simulink model "k1vistst"  (Simulink 8.5)
settings: Solver=ode45  StartTime=0.0  StopTime=10.0  RelTol=1e-3
libraries: cdsCDI64 x2, cdsCDO64 x2, cdsEpicsBinIn x2, cdsAdcx0 x1, dac x1, TYPEBP_MASTER x1, cdsBit2Word x1, cdsWord2Bit x1, cdsParameters x1
settings Model: Creator=keiko  LastModifiedBy=controls
settings DataIOCC: SignalLoggingSaveFormat=Dataset
settings OptimizationCC: ExpressionDepthLimit=128
settings DebuggingCC: UnderspecifiedInitializationDetection=Simplified  MergeDetectMultiDrivingBlocksExec=error  SolverPrmCheckMsg=warning  FcnCallInpInsideContextMsg=EnableAllAsError  StateNameClashWarn=none
settings GRTTargetCC: CombineOutputUpdateFcns=on  GRTInterface=off

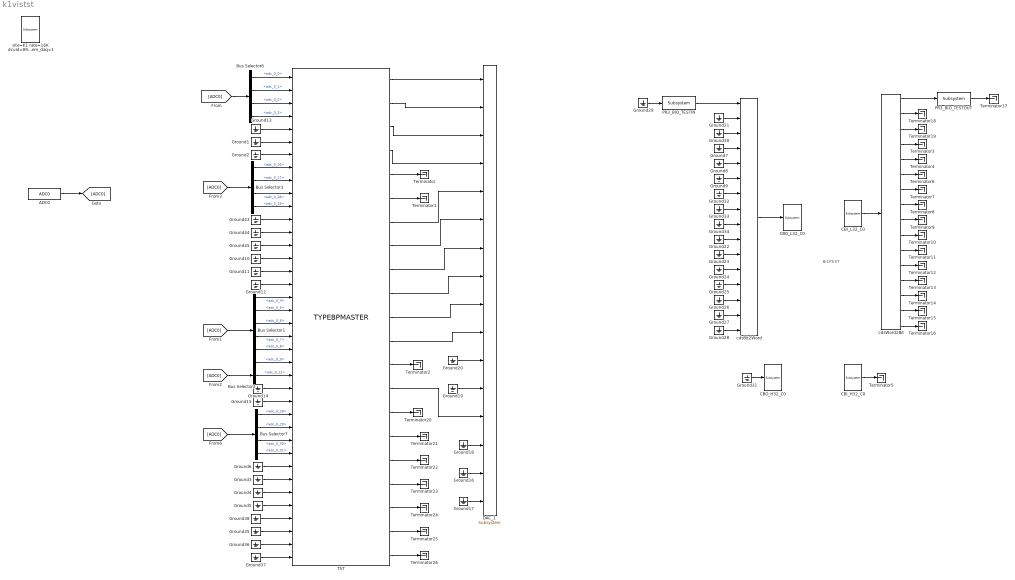
== system k1vistst ==
  note: BIOTEST
  ADC0 : cdsAdcx0/ADC0  Tag=cdsAdc  Description=|
      | type-GSC_16AI64SSA
      | card_num=0
      settings: AttributesFormatString=%<Description>\n%<Tag>
  Bus Selector1 : BusSelector  Description=ADC Selector  OutputSignals=adc_0_4,adc_0_5,adc_0_6,adc_0_7,adc_0_8,adc_0_9
      settings: AttributesFormatString=%<Description>
  Bus Selector2 : BusSelector  Description=ADC Selector  OutputSignals=adc_0_12
      settings: AttributesFormatString=%<Description>
  Bus Selector3 : BusSelector  Description=ADC Selector  OutputSignals=adc_0_16,adc_0_17,adc_0_18,adc_0_19
      settings: AttributesFormatString=%<Description>
  Bus Selector6 : BusSelector  Description=ADC Selector  OutputSignals=adc_0_0,adc_0_1,adc_0_2,adc_0_3
      settings: AttributesFormatString=%<Description>
  Bus Selector7 : BusSelector  Description=ADC Selector  OutputSignals=adc_0_28,adc_0_29,adc_0_30,adc_0_31
      settings: AttributesFormatString=%<Description>
  CBI_H32_C0 : cdsCDI64/Subsystem  Tag=cdsCDI64  Description=card_num=1
      settings: AttributesFormatString=%<Tag>\n%<Description>
  CBI_L32_C0 : cdsCDI64/Subsystem  Tag=cdsCDI64  Description=card_num=0
      settings: AttributesFormatString=%<Tag>\n%<Description>
  CBO_H32_C0 : cdsCDO64/Subsystem  Tag=cdsCDO64  Description=card_num=1
      settings: AttributesFormatString=%<Tag>\n%<Description>
  CBO_L32_C0 : cdsCDO64/Subsystem  Tag=cdsCDO64  Description=card_num=0
      settings: AttributesFormatString=%<Tag>\n%<Description>
  DAC_1 : dac/Subsystem  Description=|
      | type=GSC_16AO16,
      | card_num=0
      settings: AttributesFormatString=%<Description>
  Ground{1..38,43..45} (41 alike) : Ground
  PR3_BIO_TESTIN : cdsEpicsBinIn/Subsystem  Tag=cdsEpicsBinIn  Description=|
      | Purpose:                                                                            
      | Create an EPICS binary (0 or 1) input channel to the FE realtime controls.          
      |                                                                                     
      | Operation:                                                                          
      | Outputs value from an EPICS ai record. Value is binary input (bi Epics record type).
      |                                                                                     
      | Usage:                                                                              
      | Name the part with the desired EPICS channel name.
      settings: AttributesFormatString=%<Tag>
  PR3_BIO_TESTOUT : cdsEpicsBinIn/Subsystem  Tag=cdsEpicsBinIn  Description=|
      | Purpose:                                                                            
      | Create an EPICS binary (0 or 1) input channel to the FE realtime controls.          
      |                                                                                     
      | Operation:                                                                          
      | Outputs value from an EPICS ai record. Value is binary input (bi Epics record type).
      |                                                                                     
      | Usage:                                                                              
      | Name the part with the desired EPICS channel name.
      settings: AttributesFormatString=%<Tag>
  TST : TYPEBP_MASTER/TYPEBPMASTER
      settings: AttributesFormatString=%<Description>
  Terminator{,1..26} (27 alike) : Terminator
  cdsBit2Word : cdsBit2Word/cdsBit2Word  Tag=cdsBit2Word  Description=Forms single 16 bit integer from 16 0/1 inputs.
      settings: AttributesFormatString=%<Tag>
  cdsWord2Bit : cdsWord2Bit/cdsWord2Bit  Tag=cdsWord2Bit  Description=Generate 16 0/1 outputs from single 16-bit integer input
      settings: AttributesFormatString=cdsWord2Bit
  site=K1 rate=16K dcuid=89 host=k1pr0 specific_cpu=4 adcSlave=1 shmem_daq=1 : cdsParameters/Subsystem  Tag=cdsParameters  Description=|
      | Purpose:                                                                                                                                                                                                                                
      | Provide system parameters to the FE code generator to properly configure the generated EPICS names, rep rate of the FE controller, and the Data Acquisition node ID for proper storage of data from this FE controller.                 
      |                                                                                                                                                                                                                                         
      | Useage:                                                                                                                                                                                                                                 
      | The part NAME field is used to identify the FE parameters. It must be of the form:                                                                                                                                                      
      | site=                                                                                                                                                                                                                                   
      | rate=                                                                                                                                                                                                                                   
      | dcuid=                                                                                                                                                                                                                                  
      |                                                                                                                                                                                                                                         
      | Where:                                                                                                                                                                                                                                  
      | site= argument may be H1, H2, L1, M1, G1, either as a single argument or multiple, for example site=H1,H2. These are the only names allowed. These will become the first two characters of all EPICS and signal names (for example G1:).
      |                                                                                                                                                                                                                                         
      | rate= may be 2K, 16K, 32K, or 64K                                                                                                                                                                                                       
      |                                                                                                                                                                                                                                         
      | dcuid= is site specific ie it must be unique at each site.
      settings: AttributesFormatString=%<Tag>
  wires:
  ADC0/1 -> [ADC0]
  [ADC0] -> Bus Selector6/1
  [ADC0] -> Bus Selector1/1
  Bus Selector6/1 -> TST/1  "<adc_0_0>"
  Bus Selector6/2 -> TST/2  "<adc_0_1>"
  Bus Selector6/3 -> TST/3  "<adc_0_2>"
  Bus Selector6/4 -> TST/4  "<adc_0_3>"
  Bus Selector3/4 -> TST/11  "<adc_0_19>"
  Ground11/1 -> TST/16
  Ground43/1 -> TST/12
  Ground2/1 -> TST/7
  Ground44/1 -> TST/13
  Ground1/1 -> TST/6
  Ground12/1 -> TST/17
  Ground13/1 -> TST/5
  Bus Selector3/1 -> TST/8  "<adc_0_16>"
  Bus Selector3/3 -> TST/10  "<adc_0_18>"
  Bus Selector3/2 -> TST/9  "<adc_0_17>"
  Ground10/1 -> TST/15
  Ground45/1 -> TST/14
  Bus Selector1/1 -> TST/18  "<adc_0_4>"
  Bus Selector1/2 -> TST/19  "<adc_0_5>"
  Bus Selector1/3 -> TST/20  "<adc_0_6>"
  Bus Selector1/4 -> TST/21  "<adc_0_7>"
  Bus Selector1/5 -> TST/22  "<adc_0_8>"
  Bus Selector1/6 -> TST/23  "<adc_0_9>"
  Ground14/1 -> TST/25
  Ground15/1 -> TST/26
  [ADC0] -> Bus Selector2/1
  Bus Selector2/1 -> TST/24  "<adc_0_12>"
  TST/2 -> DAC_1/2
  TST/3 -> DAC_1/3
  TST/4 -> DAC_1/4
  TST/7 -> DAC_1/5
  TST/8 -> DAC_1/6
  TST/9 -> DAC_1/7
  TST/10 -> DAC_1/8
  TST/14 -> DAC_1/13
  [ADC0] -> Bus Selector3/1
  TST/11 -> DAC_1/9
  TST/12 -> DAC_1/10
  Ground20/1 -> DAC_1/11
  Ground19/1 -> DAC_1/12
  Ground18/1 -> DAC_1/14
  Ground16/1 -> DAC_1/15
  Ground17/1 -> DAC_1/16
  CBI_H32_C0/1 -> Terminator5/1
  CBI_L32_C0/1 -> cdsWord2Bit/1
  Ground31/1 -> CBO_H32_C0/1
  cdsBit2Word/1 -> CBO_L32_C0/1
  PR3_BIO_TESTIN/1 -> cdsBit2Word/1
  Ground29/1 -> PR3_BIO_TESTIN/1
  Ground25/1 -> cdsBit2Word/13
  Ground24/1 -> cdsBit2Word/12
  Ground33/1 -> cdsBit2Word/8
  Ground9/1 -> cdsBit2Word/6
  Ground27/1 -> cdsBit2Word/15
  Ground21/1 -> cdsBit2Word/2
  Ground22/1 -> cdsBit2Word/10
  Ground23/1 -> cdsBit2Word/11
  Ground34/1 -> cdsBit2Word/9
  Ground8/1 -> cdsBit2Word/5
  Ground26/1 -> cdsBit2Word/14
  Ground32/1 -> cdsBit2Word/7
  Ground28/1 -> cdsBit2Word/16
  Ground7/1 -> cdsBit2Word/4
  Ground30/1 -> cdsBit2Word/3
  cdsWord2Bit/1 -> PR3_BIO_TESTOUT/1
  cdsWord2Bit/2 -> Terminator18/1
  cdsWord2Bit/3 -> Terminator19/1
  cdsWord2Bit/4 -> Terminator3/1
  cdsWord2Bit/5 -> Terminator4/1
  cdsWord2Bit/6 -> Terminator6/1
  cdsWord2Bit/7 -> Terminator7/1
  cdsWord2Bit/8 -> Terminator8/1
  cdsWord2Bit/9 -> Terminator9/1
  cdsWord2Bit/10 -> Terminator10/1
  cdsWord2Bit/11 -> Terminator11/1
  cdsWord2Bit/12 -> Terminator12/1
  cdsWord2Bit/13 -> Terminator13/1
  cdsWord2Bit/14 -> Terminator14/1
  cdsWord2Bit/15 -> Terminator15/1
  cdsWord2Bit/16 -> Terminator16/1
  PR3_BIO_TESTOUT/1 -> Terminator17/1
  TST/20 -> Terminator25/1
  TST/19 -> Terminator24/1
  TST/18 -> Terminator23/1
  TST/17 -> Terminator22/1
  TST/21 -> Terminator26/1
  TST/15 -> Terminator20/1
  Bus Selector7/2 -> TST/28  "<adc_0_29>"
  Bus Selector7/3 -> TST/29  "<adc_0_30>"
  Bus Selector7/4 -> TST/30  "<adc_0_31>"
  Ground4/1 -> TST/33
  Ground5/1 -> TST/34
  Ground3/1 -> TST/32
  Ground6/1 -> TST/31
  Ground36/1 -> TST/37
  Ground37/1 -> TST/38
  Ground35/1 -> TST/36
  Ground38/1 -> TST/35
  [ADC0] -> Bus Selector7/1
  TST/16 -> Terminator21/1
  TST/13 -> Terminator2/1
  Bus Selector7/1 -> TST/27  "<adc_0_28>"
  TST/5 -> Terminator/1
  TST/6 -> Terminator1/1
  TST/1 -> DAC_1/1
